simulink model "WMMSupportingForcesGP2021b"  (R2021b)
settings: Solver=ode23t  StartTime=0.0  StopTime=inf  FixedStep=.001  RelTol=1e-3  AbsTol=1e-3
InitFcn:
  | InitializeSimulationGP
  | SimulationParametersGP
values from neighbouring files (symbols this model uses):
  B11_r_B11C = [0.23805608; 0.13201777; 0]    [InitializeSimulationGP.m]
  B11_r_B11Tc1 = [L11; 0; 0]    [InitializeSimulationGP.m]
  B11_Rot_Tc1 = eye(3)    [InitializeSimulationGP.m]
  B11cI = [0.28426000 -0.06487287 0;         -0.06487287  0.54237481 0;                   0  0          0.67891020]    [InitializeSimulationGP.m]
  B12_r_B12C = [0.60504569; 0.27199376; 0.00002484]    [InitializeSimulationGP.m]
  B12_r_B12Tc2 = [L12;0;0]    [InitializeSimulationGP.m]
  B12_Rot_Tc2 = eye(3)    [InitializeSimulationGP.m]
  B12cI = [1.18803886 -2.36786418 0.00280315;          -2.36786418 6.31493281 0.00022322;           0.00280315 0.00022322 7.40915161]    [InitializeSimulationGP.m]
  B31_r_B31C = [0.35781210 0 0]    [InitializeSimulationGP.m]
  B31_Rot_B41 = eye(3)    [InitializeSimulationGP.m]
  B31cI = diag([0.03150902 0.90735702 0.90763033])    [InitializeSimulationGP.m]
  B32_r_B32C = [0.35781210 0 0]    [InitializeSimulationGP.m]
  B32_Rot_B42 = eye(3)    [InitializeSimulationGP.m]
  B32cI = diag([0.03150902 0.90735702 0.90763033])    [InitializeSimulationGP.m]
  B41_r_B41C = [0.55785997 0 0]    [InitializeSimulationGP.m]
  B41_r_B41Tc1 = [lc1;0;0]    [InitializeSimulationGP.m]
  B41cI = diag([0.00370720 0.55759812 0.55785997])    [InitializeSimulationGP.m]
  B42_r_B42C = [0.55785997 0 0]    [InitializeSimulationGP.m]
  B42_r_B42Tc2 = [lc2; 0; 0]    [InitializeSimulationGP.m]
  B42cI = diag([0.00370720 0.55759812 0.55785997])    [InitializeSimulationGP.m]
  B52_r_B52C = [0 0 0.56802906]    [InitializeSimulationGP.m]
  B52_r_B52P32 = [lc3; 0; 0]    [InitializeSimulationGP.m]
  B52_Rot_P32 = eye(3)    [InitializeSimulationGP.m]
  B52cI = diag([0.91789884, 0.91790043, 0.00091463])    [InitializeSimulationGP.m]
  Bc1_r_Bc1B11 = [L1; 0; 0]    [InitializeSimulationGP.m]
  Bc1_r_Bc1B31 = [0;0;0]    [InitializeSimulationGP.m]
  Bc1_r_Bc1C = [0.14178771; 0.16555780; 0]    [InitializeSimulationGP.m]
  Bc1_V = [0;0;0;0;0;0]    [InitializeSimulationGP.m]
  Bc1cI = [+5.892211080 +5.476111360 -0.000019630;          +5.476111360 +28.66965601 -0.000024550;          -0.000019630 -0.000024550 +29.78955950]    [InitializeSimulationGP.m]
  Bc2_r_Bc2B12 = [L2;0;0]    [InitializeSimulationGP.m]
  Bc2_r_Bc2B32 = [0;0;0]    [InitializeSimulationGP.m]
  Bc2_r_Bc2C = [0.54319901; 0.10543875; 0]    [InitializeSimulationGP.m]
  Bc2cI = [0.48071390 0.52924041 0;          0.52924041 5.80912352 0;              0      0          5.97255351]    [InitializeSimulationGP.m]
  BC_r_BCBM = [xCA; yCA; zCA]    [SimulationParametersGP.m]
  BC_Rot_BM = eye(3)    [SimulationParametersGP.m]
  BCI = diag([100 1200 1000])    [SimulationParametersGP.m]
  beta1 = atan2d(374.261,935)*pi/180    [InitializeSimulationGP.m]
  beta2 = atan2d(45.757,373.313)*pi/180    [InitializeSimulationGP.m]
  beta3 = atan2d(139.50,1132.19)*pi/180    [InitializeSimulationGP.m]
  beta4 = atan2d(88.061,296.198)*pi/180    [InitializeSimulationGP.m]
  betaGround = 1e6    (= 1000000)    [SimulationParametersGP.m]
  BFL = 0.05    [SimulationParametersGP.m]
  BFR = 0.05    [SimulationParametersGP.m]
  BM_r_BMBMp = [0;0;0]    [SimulationParametersGP.m]
  BM_Rot_BMp = [cos(gamma) -sin(gamma) 0; sin(gamma) cos(gamma) 0; 0 0 1]    [SimulationParametersGP.m]
  BMp_r_BMpBc1 = [0.185;0;0.205]    [InitializeSimulationGP.m]
  BMp_Rot_Bc1 = [cos(alpha1) -sin(alpha1)  0;                  0            0       -1;                sin(alpha1)  cos(alpha1)  0]    [InitializeSimulationGP.m]
  BRL = 0.05    [SimulationParametersGP.m]
  BRR = 0.05    [SimulationParametersGP.m]
  cc = 0.0    (= 0)    [SimulationParametersGP.m]
  D22F = [0;0;0;0;0;0]    [InitializeSimulationGP.m]
  dT = 0.01    [SimulationParametersGP.m]
  g0 = 9.8066    [SimulationParametersGP.m]
  ground_stiffness = 1e8    (= 100000000)    [SimulationParametersGP.m]
  l1 = 1.15-cc    (= 1.15)    [SimulationParametersGP.m]
  L1 = 1.0071227324212    (= 1.00712273242)    [InitializeSimulationGP.m]
  L11 = 0.37610632101293    (= 0.376106321013)    [InitializeSimulationGP.m]
  L12 = 0.30901132665325    (= 0.309011326653)    [InitializeSimulationGP.m]
  l2 = 1.15+cc    (= 1.15)    [SimulationParametersGP.m]
  L2 = 1.132185817991    (= 1.13218581799)    [InitializeSimulationGP.m]
  lc1 = 0.745    [InitializeSimulationGP.m]
  lc2 = 0.745    [InitializeSimulationGP.m]
  mB11 = 25.52660174    [InitializeSimulationGP.m]
  mB12 = 33.92850233    [InitializeSimulationGP.m]
  mB31 = 17.36281648    [InitializeSimulationGP.m]
  mB32 = 17.36281648    [InitializeSimulationGP.m]
  mB41 = 10.34519231    [InitializeSimulationGP.m]
  mB42 = 10.34519231    [InitializeSimulationGP.m]
  mB52 = 6.73059863    [InitializeSimulationGP.m]
  mBC = 2200    [SimulationParametersGP.m]
  mBc1 = 307.29601379    [InitializeSimulationGP.m]
  mBc2 = 54.58702836    [InitializeSimulationGP.m]
  mFL = 60    [SimulationParametersGP.m]
  mFR = 60    [SimulationParametersGP.m]
  mP22 = 9.26136143    [InitializeSimulationGP.m]
  mP32 = 570.18877059    [InitializeSimulationGP.m]
  mRR = 60    [SimulationParametersGP.m]
  mw = mFL    (= 60)    [SimulationParametersGP.m]
  P22_r_P22C = [0.62192523 0 0]    [InitializeSimulationGP.m]
  P22_Rot_B52 = eye(3)    [InitializeSimulationGP.m]
  P22cI = diag([0.00662754, 1.48387017, 1.48398069])    [InitializeSimulationGP.m]
  P32_r_P32C = [0.25466704; -0.13034397; -0.01302248]    [InitializeSimulationGP.m]
  P32_r_P32D22 = [0.40499744871392; -0.13130517281345; -0.013385243295654]    [InitializeSimulationGP.m]
  P32_Rot_D22 = [1 0 0;              0 0.9707729441837 0.23999977258512;              0 -0.23999977258512 0.9707729441837]    [InitializeSimulationGP.m]
  P32cI = [46.81220713 0.38607676 -0.00453819;          0.38607676 71.92201786 -1.14320993;          -0.00453819 -1.14320993 67.38128576]    [InitializeSimulationGP.m]
  R0FL = 0.35    [SimulationParametersGP.m]
  R0FR = 0.35    [SimulationParametersGP.m]
  R0RL = 0.35    [SimulationParametersGP.m]
  R0RR = 0.35    [SimulationParametersGP.m]
  Rw = R0FL    (= 0.35)    [SimulationParametersGP.m]
  Tc1_r_Tc1Bc2 = [0.098495302558553; 0.01838181329939; 0]    [InitializeSimulationGP.m]
  Tc1_Rot_Bc2 = [cos(alpha2) -sin(alpha2) 0;                sin(alpha2)  cos(alpha2) 0;                0            0           1]    [InitializeSimulationGP.m]
  Tc2_r_Tc2P22 = [-0.048858374920227;0.36587359346146;0.035276938723102]    [InitializeSimulationGP.m]
  Tc2_Rot_P22 = [0.95853460763586 -0.27664713597974  0.0683942111482;                0.28497614981675  0.93051946315663 -0.23004808784757;                0                 0.23999977258511  0.9707729441837]    [InitializeSimulationGP.m]
  Th1A = 10*pi/180    (= 0.174532925199)    [InitializeSimulationGP.m]
  Th1B = 20*pi/180    (= 0.349065850399)    [InitializeSimulationGP.m]
  Th1f = 1    [InitializeSimulationGP.m]
  Th2A = 15*pi/180    (= 0.261799387799)    [InitializeSimulationGP.m]
  Th2B = -70*pi/180    (= -1.2217304764)    [InitializeSimulationGP.m]
  Th2f = 2    [InitializeSimulationGP.m]
  w = wFL    (= 0.875)    [SimulationParametersGP.m]
  W_r_WBc1 = [0.185;0;0.205]    [InitializeSimulationGP.m]
  W_Rot_Bc1 = [cos(alpha1) -sin(alpha1)  0;                  0            0       -1;                sin(alpha1)  cos(alpha1)  0]    [InitializeSimulationGP.m]
  x10 = 0.83    [InitializeSimulationGP.m]
  x20 = 0.83    [InitializeSimulationGP.m]
  x3A = 0.2    [InitializeSimulationGP.m]
  x3B = 0.3    [InitializeSimulationGP.m]
  x3f = 1    [InitializeSimulationGP.m]
  xCA = 0.5    [SimulationParametersGP.m]
  xf = [1;0;0;0;0;0]    [InitializeSimulationGP.m]
  yCA = 0    [SimulationParametersGP.m]
  zC = 0.45    [SimulationParametersGP.m]
  zCA = .25    (= 0.25)    [SimulationParametersGP.m]
  ztau = [0;0;0;0;0;1]    [InitializeSimulationGP.m]
undefined symbols (not defined in the file or in its folder): alphaFL_meas, alphaFR_meas, alphaRL_meas, alphaRR_meas, B11_V, B11Ftot, B12_U_Tc2, B12_V, B12Ftot, B31_r_B31B41, B31_V, B31FTot, B32_r_B32B42, B32_U_B42, B32_V, B32FTot, B41_V, B41FTot, B42_Rot_Tc2, B42_U_Tc2, B42_V, B42FTot, B52_U_P32, B52_V, B52Ftot, Bc1Tot, Bc2_Rot_B12, Bc2_Rot_B32, Bc2_U_B12, Bc2_U_B32, Bc2_V, Bc2Tot, betaC_meas, D22_V, deltaFL_cmd, deltaFL_meas, deltaFR_cmd, deltaFR_meas, deltaRL_cmd, deltaRL_meas, deltaRR_cmd, deltaRR_meas, dOmegaFL_meas, dOmegaFR_meas, dOmegaRL_meas, dOmegaRR_meas, dPsi_meas, dq1, dq11, dq12, dq2, dq21, dq22, dx1, dx2, Floor, FTot_S1, FTot_S2P, FTot_S2R, FzFL ... (+63)
libraries: sm_lib x94, nesl_utility x63, simulink x5
(part 2 of 11)

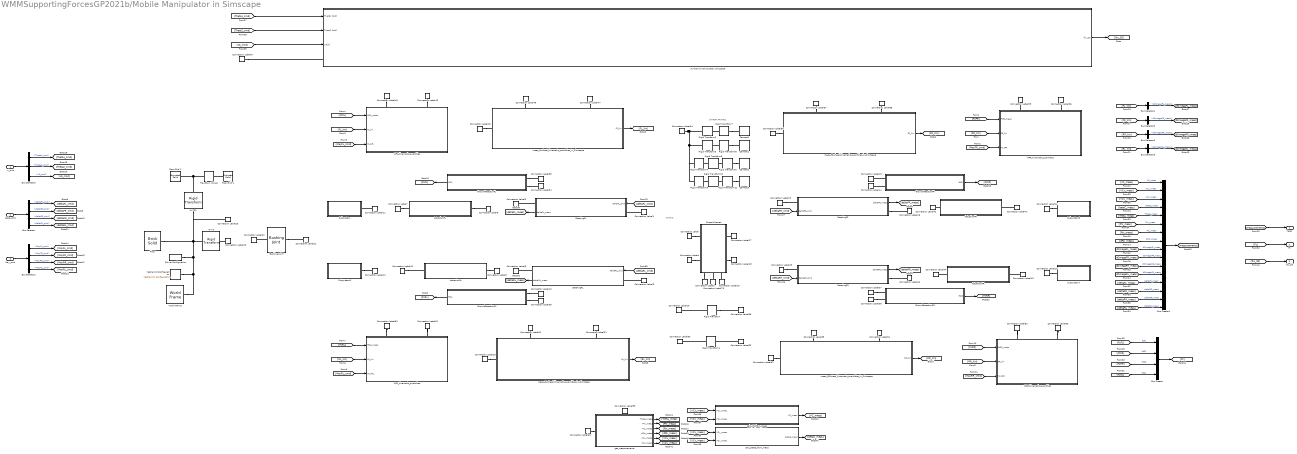
== system WMMSupportingForcesGP2021b/Mobile Manipulator in Simscape ==
  note: CAMERA FRAMES
  note: CHASIS
  xi_cmd : Inport
  delta_cmd : Inport  Port=2
  May_cmd : Inport  Port=3
  ActuationFL : Subsystem
  ActuationFR : Subsystem
  ActuationRL : Subsystem
  ActuationRR : Subsystem
  Bus Creator : BusCreator  Inputs=FzFL,FzFR,FzRR,FzRL
  Bus Creator1 : BusCreator  Inputs=VC_meas,VCx_meas,VCy_meas,betaC_meas,Theta_meas,Phi_meas,Psi_meas,dPsi_meas,dOmegaFL_meas,dOmegaFR_meas,dOmegaRR_meas,dOmegaRL_meas,deltaFL_meas,deltaFR_meas,deltaRR_meas,deltaRL_meas
  Bus Selector : BusSelector  OutputSignals=deltaFL_cmd,deltaFR_cmd,deltaRR_cmd,deltaRL_cmd
  Bus Selector1 : BusSelector  OutputSignals=MayFL_cmd,MayFR_cmd,MayRR_cmd,MayRL_cmd
  Bus Selector2 : BusSelector  OutputSignals=Theta1_cmd,Theta2_cmd,x3_cmd
  Bus Selector3 : BusSelector  OutputSignals=dOmegaFR_meas
  Bus Selector4 : BusSelector  OutputSignals=dOmegaFL_meas
  Bus Selector5 : BusSelector  OutputSignals=dOmegaRR_meas
  Bus Selector6 : BusSelector  OutputSignals=dOmegaRL_meas
  Bushing Joint : sm_lib/Joints/Bushing Joint  JointMode=Normal  SenseConstraintForce=off  SenseConstraintForceX=off  SenseConstraintForceY=off  SenseConstraintForceZ=off  SenseConstraintTorque=off  SenseConstraintTorqueX=off  SenseConstraintTorqueY=off  SenseConstraintTorqueZ=off  SenseTotalForce=off  SenseTotalForceX=off  SenseTotalForceY=off  SenseTotalForceZ=off  SenseTotalTorque=off  SenseTotalTorqueX=off  SenseTotalTorqueY=off  SenseTotalTorqueZ=off  CompositeWrenchDir=FollowerOnBase  CompositeWrenchFrame=BaseFrame  PxEquilibriumPosition=0  PxEquilibriumPositionUnits=m  PxSpringStiffness=0  PxSpringStiffnessUnits=N/m  PxDampingCoefficient=0  PxDampingCoefficientUnits=N/(m/s)  PxTorqueActuationMode=NoTorque  PxMotionActuationMode=ComputedMotion  PxSensePosition=off  PxSenseVelocity=off  PxSenseAcceleration=off  PxSenseTorqueForce=off  PxSenseLowerLimitTorqueForce=off  PxSenseUpperLimitTorqueForce=off  PxLowerLimitSpecify=off  PxLowerLimitBound=-1  PxLowerLimitBoundUnits=m  PxLowerLimitStiffness=1e6  PxLowerLimitStiffnessUnits=N/m  PxLowerLimitDamping=1e3  PxLowerLimitDampingUnits=N/(m/s)  PxLowerLimitTransitionRegionWidth=1e-4  PxLowerLimitTransitionRegionWidthUnits=m  PxUpperLimitSpecify=off  PxUpperLimitBound=1  PxUpperLimitBoundUnits=m  PxUpperLimitStiffness=1e6  PxUpperLimitStiffnessUnits=N/m  PxUpperLimitDamping=1e3  PxUpperLimitDampingUnits=N/(m/s)  PxUpperLimitTransitionRegionWidth=1e-4  PxUpperLimitTransitionRegionWidthUnits=m  PxPositionTargetSpecify=off  PxPositionTargetPriority=High  PxPositionTargetValue=0  PxPositionTargetValueUnits=m  PxVelocityTargetSpecify=off  PxVelocityTargetPriority=High  PxVelocityTargetValue=0  PxVelocityTargetValueUnits=m/s  PyEquilibriumPosition=0  PyEquilibriumPositionUnits=m  PySpringStiffness=0  PySpringStiffnessUnits=N/m  PyDampingCoefficient=0  PyDampingCoefficientUnits=N/(m/s)  PyTorqueActuationMode=NoTorque  PyMotionActuationMode=ComputedMotion  PySensePosition=off  PySenseVelocity=off  PySenseAcceleration=off  PySenseTorqueForce=off  PySenseLowerLimitTorqueForce=off  PySenseUpperLimitTorqueForce=off  PyLowerLimitSpecify=off  PyLowerLimitBound=-1  PyLowerLimitBoundUnits=m  PyLowerLimitStiffness=1e6  PyLowerLimitStiffnessUnits=N/m  PyLowerLimitDamping=1e3  PyLowerLimitDampingUnits=N/(m/s)  PyLowerLimitTransitionRegionWidth=1e-4  PyLowerLimitTransitionRegionWidthUnits=m  PyUpperLimitSpecify=off  PyUpperLimitBound=1  PyUpperLimitBoundUnits=m  PyUpperLimitStiffness=1e6  PyUpperLimitStiffnessUnits=N/m  PyUpperLimitDamping=1e3  PyUpperLimitDampingUnits=N/(m/s)  PyUpperLimitTransitionRegionWidth=1e-4  PyUpperLimitTransitionRegionWidthUnits=m  PyPositionTargetSpecify=off  PyPositionTargetPriority=High  PyPositionTargetValue=0  PyPositionTargetValueUnits=m  PyVelocityTargetSpecify=off  PyVelocityTargetPriority=High  PyVelocityTargetValue=0  PyVelocityTargetValueUnits=m/s  PzEquilibriumPosition=0  PzEquilibriumPositionUnits=m  PzSpringStiffness=0  PzSpringStiffnessUnits=N/m  PzDampingCoefficient=0  PzDampingCoefficientUnits=N/(m/s)  PzTorqueActuationMode=NoTorque  PzMotionActuationMode=ComputedMotion  PzSensePosition=off  PzSenseVelocity=off  PzSenseAcceleration=off  PzSenseTorqueForce=off  PzSenseLowerLimitTorqueForce=off  PzSenseUpperLimitTorqueForce=off  PzLowerLimitSpecify=off  PzLowerLimitBound=-1  PzLowerLimitBoundUnits=m  PzLowerLimitStiffness=1e6  PzLowerLimitStiffnessUnits=N/m  PzLowerLimitDamping=1e3  PzLowerLimitDampingUnits=N/(m/s)  PzLowerLimitTransitionRegionWidth=1e-4  PzLowerLimitTransitionRegionWidthUnits=m  PzUpperLimitSpecify=off  PzUpperLimitBound=1  PzUpperLimitBoundUnits=m  PzUpperLimitStiffness=1e6  PzUpperLimitStiffnessUnits=N/m  PzUpperLimitDamping=1e3  PzUpperLimitDampingUnits=N/(m/s)  PzUpperLimitTransitionRegionWidth=1e-4  PzUpperLimitTransitionRegionWidthUnits=m  PzPositionTargetSpecify=off  PzPositionTargetPriority=High  PzPositionTargetValue=0  PzPositionTargetValueUnits=m  PzVelocityTargetSpecify=off  PzVelocityTargetPriority=High  PzVelocityTargetValue=0  PzVelocityTargetValueUnits=m/s  RxEquilibriumPosition=0  RxEquilibriumPositionUnits=deg  RxSpringStiffness=0  RxSpringStiffnessUnits=N*m/deg  RxDampingCoefficient=0  RxDampingCoefficientUnits=N*m/(deg/s)  RxTorqueActuationMode=NoTorque  RxMotionActuationMode=ComputedMotion  RxSensePosition=off  RxSenseVelocity=off  RxSenseAcceleration=off  RxSenseTorqueForce=off  RxSenseLowerLimitTorqueForce=off  RxSenseUpperLimitTorqueForce=off  RxLowerLimitSpecify=off  RxLowerLimitBound=-90  RxLowerLimitBoundUnits=deg  RxLowerLimitStiffness=1e4  RxLowerLimitStiffnessUnits=N*m/deg  RxLowerLimitDamping=10  RxLowerLimitDampingUnits=N*m/(deg/s)  RxLowerLimitTransitionRegionWidth=0.1  RxLowerLimitTransitionRegionWidthUnits=deg  RxUpperLimitSpecify=off  RxUpperLimitBound=90  RxUpperLimitBoundUnits=deg  RxUpperLimitStiffness=1e4  RxUpperLimitStiffnessUnits=N*m/deg  RxUpperLimitDamping=10  RxUpperLimitDampingUnits=N*m/(deg/s)  RxUpperLimitTransitionRegionWidth=0.1  RxUpperLimitTransitionRegionWidthUnits=deg  RxPositionTargetSpecify=off  RxPositionTargetPriority=High  RxPositionTargetValue=0  RxPositionTargetValueUnits=deg  RxVelocityTargetSpecify=off  RxVelocityTargetPriority=High  RxVelocityTargetValue=0  RxVelocityTargetValueUnits=deg/s  RyEquilibriumPosition=0  RyEquilibriumPositionUnits=deg  RySpringStiffness=0  RySpringStiffnessUnits=N*m/deg  RyDampingCoefficient=0  RyDampingCoefficientUnits=N*m/(deg/s)  RyTorqueActuationMode=NoTorque  RyMotionActuationMode=ComputedMotion  RySensePosition=off  RySenseVelocity=off  RySenseAcceleration=off  RySenseTorqueForce=off  RySenseLowerLimitTorqueForce=off  RySenseUpperLimitTorqueForce=off  RyLowerLimitSpecify=off  RyLowerLimitBound=-90  RyLowerLimitBoundUnits=deg  RyLowerLimitStiffness=1e4  RyLowerLimitStiffnessUnits=N*m/deg  RyLowerLimitDamping=10  RyLowerLimitDampingUnits=N*m/(deg/s)  RyLowerLimitTransitionRegionWidth=0.1  RyLowerLimitTransitionRegionWidthUnits=deg  RyUpperLimitSpecify=off  RyUpperLimitBound=90  RyUpperLimitBoundUnits=deg  RyUpperLimitStiffness=1e4  RyUpperLimitStiffnessUnits=N*m/deg  RyUpperLimitDamping=10  RyUpperLimitDampingUnits=N*m/(deg/s)  RyUpperLimitTransitionRegionWidth=0.1  RyUpperLimitTransitionRegionWidthUnits=deg  RyPositionTargetSpecify=off  RyPositionTargetPriority=High  RyPositionTargetValue=0  RyPositionTargetValueUnits=deg  RyVelocityTargetSpecify=off  RyVelocityTargetPriority=High  RyVelocityTargetValue=0  RyVelocityTargetValueUnits=deg/s  RzEquilibriumPosition=0  RzEquilibriumPositionUnits=deg  RzSpringStiffness=0  RzSpringStiffnessUnits=N*m/deg  RzDampingCoefficient=0  RzDampingCoefficientUnits=N*m/(deg/s)  RzTorqueActuationMode=NoTorque  RzMotionActuationMode=ComputedMotion  RzSensePosition=off  RzSenseVelocity=off  RzSenseAcceleration=off  RzSenseTorqueForce=off  RzSenseLowerLimitTorqueForce=off  RzSenseUpperLimitTorqueForce=off  RzLowerLimitSpecify=off  RzLowerLimitBound=-90  RzLowerLimitBoundUnits=deg  RzLowerLimitStiffness=1e4  RzLowerLimitStiffnessUnits=N*m/deg  RzLowerLimitDamping=10  RzLowerLimitDampingUnits=N*m/(deg/s)  RzLowerLimitTransitionRegionWidth=0.1  RzLowerLimitTransitionRegionWidthUnits=deg  RzUpperLimitSpecify=off  RzUpperLimitBound=90  RzUpperLimitBoundUnits=deg  RzUpperLimitStiffness=1e4  RzUpperLimitStiffnessUnits=N*m/deg  RzUpperLimitDamping=10  RzUpperLimitDampingUnits=N*m/(deg/s)  RzUpperLimitTransitionRegionWidth=0.1  RzUpperLimitTransitionRegionWidthUnits=deg  RzPositionTargetSpecify=off  RzPositionTargetPriority=High  RzPositionTargetValue=0  RzPositionTargetValueUnits=deg  RzVelocityTargetSpecify=off  RzVelocityTargetPriority=High  RzVelocityTargetValue=0  RzVelocityTargetValueUnits=deg/s
  Camera{0..3} (4 alike) : sm_lib/Frames and Transforms/Reference Frame
  Chassis frames : Subsystem
      settings: PortSchema="{\"entries\":[{\"content\":{\"sides\":[{\"content\":{\"connectorIds\":[\"LConn1\",\"LConn2\"]},\"type\":\"ConnectorPlacement.EquallySpacedRectSide\",\"uuid\":\"eef62e1d-15c3-48f9-a200-1ec7cba34bfd\"},{\"content\":{\"connectorIds\":[\"RConn1\",\"RConn2\"],\"side\":\"RIGHT\"},\"type\":\"ConnectorPlacement.EquallySpacedRectSide\",\"uuid\":\"68cd7829-07b7-4c33-9669-dcec97cc4467\"},{\"content\":{\"connectorIds\":[],\"side\":\"TOP\"},\"type\":\"ConnectorPlacement.EquallySpacedRectSide\",\"uuid\":\"a2020256-aba7-4d86-a2a6-b0271002a0c7\"},{\"content\":{\"connectorIds\":[\"RConn3\",\"RConn4\",\"RConn5\"],\"side\":\"BOTTOM\"},\"type\":\"ConnectorPlacement.EquallySpacedRectSide\",\"uuid\":\"c369bc44-4007-4272-b5f0-3026cf2c22ef\"}]},\"type\":\"ConnectorPlacement.EquallySpacedConnector\",\"uuid\":\"d60cd83d-8810-499d-88ee-1107911897a7\"}],\"packageUris\":[\"http://schema.mathworks.com/mf0/Connector/R2020b\"],\"version\":\"1.0\"}"
  Connection Label : ConnectionLabel  Label=CFL
  Connection Label1 : ConnectionLabel  Label=CFL
  Connection Label{10,12,31,51} (4 alike) : ConnectionLabel  Label=WRLp
  Connection Label{7,11,47,49} (4 alike) : ConnectionLabel  Label=WFLp
  Connection Label{13,23,29,32,37,39,45,54,56,63} (10 alike) : ConnectionLabel  Label=W
  Connection Label{14,16,35,42,57} (5 alike) : ConnectionLabel  Label=WFR
  Connection Label15 : ConnectionLabel  Label=CFR
  Connection Label17 : ConnectionLabel  Label=CFR
  Connection Label18 : ConnectionLabel  Label=CRR
  Connection Label19 : ConnectionLabel  Label=B
  Connection Label2 : ConnectionLabel  Label=BC
  Connection Label20 : ConnectionLabel  Label=BC
  Connection Label21 : ConnectionLabel  Label=O
  Connection Label22 : ConnectionLabel  Label=S
  Connection Label{24,36,41,65} (4 alike) : ConnectionLabel  Label=WFRp
  Connection Label25 : ConnectionLabel  Label=CRR
  Connection Label{26,33,38,44,52} (5 alike) : ConnectionLabel  Label=WRR
  Connection Label{27,34,43,53} (4 alike) : ConnectionLabel  Label=WRRp
  Connection Label28 : ConnectionLabel  Label=S
  Connection Label3 : ConnectionLabel  Label=CRL
  Connection Label{6,9,30,40,50} (5 alike) : ConnectionLabel  Label=WRL
  Connection Label4 : ConnectionLabel  Label=CRL
  Connection Label{5,8,46,48,55} (5 alike) : ConnectionLabel  Label=WFL
  Connection Label58 : ConnectionLabel  Label=BM
  Connection Label59 : ConnectionLabel  Label=BC
  Connection Label60 : ConnectionLabel  Label=BM
  Connection Label62 : ConnectionLabel  Label=BMp
  Connection Label64 : ConnectionLabel  Label=BM
  Connection Label67 : ConnectionLabel  Label=BMp
  Connection Label75 : ConnectionLabel  Label=O
  Floor : sm_lib/Body Elements/Brick Solid  GraphicAmbientColor=[0.15 0.15 0.15 1.0]  BasedOnType=Density  BrickDimensions=[1000 1000 .1]  BrickDimensionUnits=m  CenterOfMass=[0 0 0]  CenterOfMassUnits=m  GraphicDiffuseColor=[0.8 1.0 0.8]  Density=1000  DensityUnits=kg/m^3  DoExposeReferenceFrame=off  GraphicEmissiveColor=[0.0 0.0 0.0 1.0]  ExportEntireGeometry=off  SerializedFrames=<Frames><Frame><Id>Frame2</Id><Value><Name>W</Name><Origin><Source>GeometricFeature</Source><FeatureName>+z -x curve</FeatureName></Origin><PrimaryAxis><DefinedDirection>+Z</DefinedDirection><Source>ReferenceFrame</Source><SourceDirection>+Z</SourceDirection><FeatureName></FeatureName></PrimaryAxis><SecondaryAxis><DefinedDirection>+X</DefinedDirection><Source>ReferenceFrame</Source><SourceDirection>+X</SourceDirection><FeatureName></FeatureName></SecondaryAxis></Value></Frame></Frames>  MarkerShape=Sphere  MarkerSize=10  GraphicType=FromGeometry  InertiaType=CalculateFromGeometry  Mass=1  MassUnits=kg  MomentsOfInertia=[1 1 1]  MomentsOfInertiaUnits=kg*m^2  GraphicOpacity=1  ProductsOfInertia=[0 0 0]  ProductsOfInertiaUnits=kg*m^2  GraphicShininess=75  GraphicSpecularColor=[0.5 0.5 0.5 1.0]  GraphicVisPropType=SimpleVisualProperties
  Floor Grid 1 : sm_lib/Body Elements/Extruded Solid  GraphicAmbientColor=[0.15 0.15 0.15 1.0]  BasedOnType=Density  CenterOfMass=[0 0 0]  CenterOfMassUnits=m  GraphicDiffuseColor=[1.0 0.2 0.4]  ExportConvexHullGeometry=off  ExtrusionCrossSection=Grid.extr_data  ExtrusionCrossSectionUnits=m  Density=1000  DensityUnits=kg/m^3  DoExposeReferenceFrame=on  GraphicEmissiveColor=[0.0 0.0 0.0 1.0]  ExportEntireGeometry=off  ExtrusionLength=Floor.h*1.005  ExtrusionLengthUnits=m  ExtrusionType=General  SerializedFrames=<Frames/>  MarkerShape=Sphere  MarkerSize=10  GraphicType=FromGeometry  InertiaType=PointMass  Mass=1  MassUnits=kg  MomentsOfInertia=[1 1 1]  MomentsOfInertiaUnits=kg*m^2  PolygonNumSides=3  GraphicOpacity=1.0  PolygonOuterRadius=1  PolygonOuterRadiusUnits=m  ProductsOfInertia=[1 1 1]  ProductsOfInertiaUnits=kg*m^2  GraphicShininess=75  GraphicSpecularColor=[0.5 0.5 0.5 1.0]  GraphicVisPropType=SimpleVisualProperties
  Floor Grid 2 : sm_lib/Body Elements/Extruded Solid  GraphicAmbientColor=[0.15 0.15 0.15 1.0]  BasedOnType=Density  CenterOfMass=[0 0 0]  CenterOfMassUnits=m  GraphicDiffuseColor=[1.0 0.0 0.2]  ExportConvexHullGeometry=off  ExtrusionCrossSection=Grid.extr_data  ExtrusionCrossSectionUnits=m  Density=1000  DensityUnits=kg/m^3  DoExposeReferenceFrame=on  GraphicEmissiveColor=[0.0 0.0 0.0 1.0]  ExportEntireGeometry=off  ExtrusionLength=Floor.h*1.005  ExtrusionLengthUnits=m  ExtrusionType=General  SerializedFrames=<Frames/>  MarkerShape=Sphere  MarkerSize=10  GraphicType=FromGeometry  InertiaType=PointMass  Mass=1  MassUnits=kg  MomentsOfInertia=[1 1 1]  MomentsOfInertiaUnits=kg*m^2  PolygonNumSides=3  GraphicOpacity=1.0  PolygonOuterRadius=1  PolygonOuterRadiusUnits=m  ProductsOfInertia=[1 1 1]  ProductsOfInertiaUnits=kg*m^2  GraphicShininess=75  GraphicSpecularColor=[0.5 0.5 0.5 1.0]  GraphicVisPropType=SimpleVisualProperties
  GroundReactionFL : Subsystem
      settings: PortSchema="{\"entries\":[{\"content\":{\"sides\":[{\"content\":{\"connectorIds\":[\"Out1\"]},\"type\":\"ConnectorPlacement.EquallySpacedRectSide\",\"uuid\":\"83a50a17-2c26-4437-a264-c8e6d16b5f5b\"},{\"content\":{\"connectorIds\":[\"RConn1\",\"RConn2\"],\"side\":\"RIGHT\"},\"type\":\"ConnectorPlacement.EquallySpacedRectSide\",\"uuid\":\"9399cf75-3dd9-45fa-85d6-db5b88096a02\"},{\"content\":{\"connectorIds\":[],\"side\":\"TOP\"},\"type\":\"ConnectorPlacement.EquallySpacedRectSide\",\"uuid\":\"59849b12-7527-4fe3-9ac1-a960d161aef4\"},{\"content\":{\"connectorIds\":[],\"side\":\"BOTTOM\"},\"type\":\"ConnectorPlacement.EquallySpacedRectSide\",\"uuid\":\"c578aa5d-499f-4dfc-8d0b-42fb5daa91e6\"}]},\"type\":\"ConnectorPlacement.EquallySpacedConnector\",\"uuid\":\"74a78a0d-1728-4273-b294-ce3cbd63255e\"}],\"packageUris\":[\"http://schema.mathworks.com/mf0/Connector/R2020b\"],\"version\":\"1.0\"}"
  GroundReactionFR : Subsystem
      settings: PortSchema="{\"entries\":[{\"content\":{\"sides\":[{\"content\":{\"connectorIds\":[\"Out1\"]},\"type\":\"ConnectorPlacement.EquallySpacedRectSide\",\"uuid\":\"83a50a17-2c26-4437-a264-c8e6d16b5f5b\"},{\"content\":{\"connectorIds\":[\"RConn1\",\"RConn2\"],\"side\":\"RIGHT\"},\"type\":\"ConnectorPlacement.EquallySpacedRectSide\",\"uuid\":\"9399cf75-3dd9-45fa-85d6-db5b88096a02\"},{\"content\":{\"connectorIds\":[],\"side\":\"TOP\"},\"type\":\"ConnectorPlacement.EquallySpacedRectSide\",\"uuid\":\"59849b12-7527-4fe3-9ac1-a960d161aef4\"},{\"content\":{\"connectorIds\":[],\"side\":\"BOTTOM\"},\"type\":\"ConnectorPlacement.EquallySpacedRectSide\",\"uuid\":\"c578aa5d-499f-4dfc-8d0b-42fb5daa91e6\"}]},\"type\":\"ConnectorPlacement.EquallySpacedConnector\",\"uuid\":\"74a78a0d-1728-4273-b294-ce3cbd63255e\"}],\"packageUris\":[\"http://schema.mathworks.com/mf0/Connector/R2020b\"],\"version\":\"1.0\"}"
  GroundReactionRL : Subsystem
      settings: PortSchema="{\"entries\":[{\"content\":{\"sides\":[{\"content\":{\"connectorIds\":[\"Out1\"]},\"type\":\"ConnectorPlacement.EquallySpacedRectSide\",\"uuid\":\"83a50a17-2c26-4437-a264-c8e6d16b5f5b\"},{\"content\":{\"connectorIds\":[\"RConn1\",\"RConn2\"],\"side\":\"RIGHT\"},\"type\":\"ConnectorPlacement.EquallySpacedRectSide\",\"uuid\":\"9399cf75-3dd9-45fa-85d6-db5b88096a02\"},{\"content\":{\"connectorIds\":[],\"side\":\"TOP\"},\"type\":\"ConnectorPlacement.EquallySpacedRectSide\",\"uuid\":\"59849b12-7527-4fe3-9ac1-a960d161aef4\"},{\"content\":{\"connectorIds\":[],\"side\":\"BOTTOM\"},\"type\":\"ConnectorPlacement.EquallySpacedRectSide\",\"uuid\":\"c578aa5d-499f-4dfc-8d0b-42fb5daa91e6\"}]},\"type\":\"ConnectorPlacement.EquallySpacedConnector\",\"uuid\":\"74a78a0d-1728-4273-b294-ce3cbd63255e\"}],\"packageUris\":[\"http://schema.mathworks.com/mf0/Connector/R2020b\"],\"version\":\"1.0\"}"
  GroundReactionRR : Subsystem
      settings: PortSchema="{\"entries\":[{\"content\":{\"sides\":[{\"content\":{\"connectorIds\":[\"Out1\"]},\"type\":\"ConnectorPlacement.EquallySpacedRectSide\",\"uuid\":\"83a50a17-2c26-4437-a264-c8e6d16b5f5b\"},{\"content\":{\"connectorIds\":[\"RConn1\",\"RConn2\"],\"side\":\"RIGHT\"},\"type\":\"ConnectorPlacement.EquallySpacedRectSide\",\"uuid\":\"9399cf75-3dd9-45fa-85d6-db5b88096a02\"},{\"content\":{\"connectorIds\":[],\"side\":\"TOP\"},\"type\":\"ConnectorPlacement.EquallySpacedRectSide\",\"uuid\":\"59849b12-7527-4fe3-9ac1-a960d161aef4\"},{\"content\":{\"connectorIds\":[],\"side\":\"BOTTOM\"},\"type\":\"ConnectorPlacement.EquallySpacedRectSide\",\"uuid\":\"c578aa5d-499f-4dfc-8d0b-42fb5daa91e6\"}]},\"type\":\"ConnectorPlacement.EquallySpacedConnector\",\"uuid\":\"74a78a0d-1728-4273-b294-ce3cbd63255e\"}],\"packageUris\":[\"http://schema.mathworks.com/mf0/Connector/R2020b\"],\"version\":\"1.0\"}"
  "Hydraulic manipulator, Simscape" : Subsystem
  MechanismConfiguration : sm_lib/Utilities/Mechanism Configuration  UniformGravity=Constant  GravityVector=[0 0 -9.8066]  GravityUnits=m/s^2  LinearizationDelta=0.001  JointModeTransitionNonlinearIterations=2
  Rigid Transform : sm_lib/Frames and Transforms/Rigid Transform  TranslationMethod=Cartesian  TranslationStandardOffset=0.3  TranslationLengthUnit=m  TranslationStandardAxis=+X  TranslationCartesianOffset=[xCA yCA zCA]  TranslationROffset=0  TranslationROffsetUnits=m  TranslationZOffset=0  TranslationZOffsetUnits=m  TranslationThetaOffset=0  TranslationThetaOffsetUnits=deg  RotationMethod=StandardAxis  RotationAngleUnits=deg  RotationStandardAxis=+Z  RotationAngle=0  RotationArbitraryAxis=[0 0 1]  FollAlignAxisA=+X  BaseAlignAxisA=+Y  FollAlignAxisB=+Y  BaseAlignAxisB=+Z  RotationSequenceAxes=FollowerAxes  RotationSequence=XYX  RotationSequenceAngles=[0 0 0]  RotationSequenceAnglesUnits=deg  RotationMatrix=[1 0 0; 0 1 0; 0 0 1]
  Rigid Transform1 : sm_lib/Frames and Transforms/Rigid Transform  TranslationMethod=None  TranslationStandardOffset=0  TranslationLengthUnit=m  TranslationStandardAxis=+Z  TranslationCartesianOffset=[0 0 0]  TranslationROffset=0  TranslationROffsetUnits=m  TranslationZOffset=0  TranslationZOffsetUnits=m  TranslationThetaOffset=0  TranslationThetaOffsetUnits=deg  RotationMethod=StandardAxis  RotationAngleUnits=rad  RotationStandardAxis=+Z  RotationAngle=gamma  RotationArbitraryAxis=[0 0 1]  FollAlignAxisA=+X  BaseAlignAxisA=+Y  FollAlignAxisB=+Y  BaseAlignAxisB=+Z  RotationSequenceAxes=FollowerAxes  RotationSequence=XYX  RotationSequenceAngles=[0 0 0]  RotationSequenceAnglesUnits=deg  RotationMatrix=[1 0 0; 0 1 0; 0 0 1]
  Rigid Transform10 : sm_lib/Frames and Transforms/Rigid Transform  TranslationMethod=None  TranslationStandardOffset=-10  TranslationLengthUnit=m  TranslationStandardAxis=+Y  TranslationCartesianOffset=[0 0 0]  TranslationROffset=0  TranslationROffsetUnits=m  TranslationZOffset=0  TranslationZOffsetUnits=m  TranslationThetaOffset=0  TranslationThetaOffsetUnits=deg  RotationMethod=StandardAxis  RotationAngleUnits=deg  RotationStandardAxis=+Z  RotationAngle=20  RotationArbitraryAxis=[0 0 1]  FollAlignAxisA=+X  BaseAlignAxisA=+Y  FollAlignAxisB=+Y  BaseAlignAxisB=+Z  RotationSequenceAxes=FollowerAxes  RotationSequence=XYX  RotationSequenceAngles=[0 0 0]  RotationSequenceAnglesUnits=deg  RotationMatrix=[1 0 0; 0 1 0; 0 0 1]
  Rigid Transform11 : sm_lib/Frames and Transforms/Rigid Transform  TranslationMethod=None  TranslationStandardOffset=-10  TranslationLengthUnit=m  TranslationStandardAxis=+Y  TranslationCartesianOffset=[0 0 0]  TranslationROffset=0  TranslationROffsetUnits=m  TranslationZOffset=0  TranslationZOffsetUnits=m  TranslationThetaOffset=0  TranslationThetaOffsetUnits=deg  RotationMethod=StandardAxis  RotationAngleUnits=deg  RotationStandardAxis=+Y  RotationAngle=20  RotationArbitraryAxis=[0 0 1]  FollAlignAxisA=+X  BaseAlignAxisA=+Y  FollAlignAxisB=+Y  BaseAlignAxisB=+Z  RotationSequenceAxes=FollowerAxes  RotationSequence=XYX  RotationSequenceAngles=[0 0 0]  RotationSequenceAnglesUnits=deg  RotationMatrix=[1 0 0; 0 1 0; 0 0 1]
  Rigid Transform2 : sm_lib/Frames and Transforms/Rigid Transform  TranslationMethod=Cartesian  TranslationStandardOffset=7  TranslationLengthUnit=m  TranslationStandardAxis=+X  TranslationCartesianOffset=[10 0 5]  TranslationROffset=0  TranslationROffsetUnits=m  TranslationZOffset=0  TranslationZOffsetUnits=m  TranslationThetaOffset=0  TranslationThetaOffsetUnits=deg  RotationMethod=None  RotationAngleUnits=deg  RotationStandardAxis=+Z  RotationAngle=0.0  RotationArbitraryAxis=[0 0 1]  FollAlignAxisA=+X  BaseAlignAxisA=+Y  FollAlignAxisB=+Y  BaseAlignAxisB=+Z  RotationSequenceAxes=FollowerAxes  RotationSequence=XYX  RotationSequenceAngles=[0 0 0]  RotationSequenceAnglesUnits=deg  RotationMatrix=[1 0 0; 0 1 0; 0 0 1]
  Rigid Transform3 : sm_lib/Frames and Transforms/Rigid Transform  TranslationMethod=Cartesian  TranslationStandardOffset=-10  TranslationLengthUnit=m  TranslationStandardAxis=+X  TranslationCartesianOffset=[-10 0 5]  TranslationROffset=0  TranslationROffsetUnits=m  TranslationZOffset=0  TranslationZOffsetUnits=m  TranslationThetaOffset=0  TranslationThetaOffsetUnits=deg  RotationMethod=None  RotationAngleUnits=deg  RotationStandardAxis=+Z  RotationAngle=0.0  RotationArbitraryAxis=[0 0 1]  FollAlignAxisA=+X  BaseAlignAxisA=+Y  FollAlignAxisB=+Y  BaseAlignAxisB=+Z  RotationSequenceAxes=FollowerAxes  RotationSequence=XYX  RotationSequenceAngles=[0 0 0]  RotationSequenceAnglesUnits=deg  RotationMatrix=[1 0 0; 0 1 0; 0 0 1]
  Rigid Transform4 : sm_lib/Frames and Transforms/Rigid Transform  TranslationMethod=Cartesian  TranslationStandardOffset=-10  TranslationLengthUnit=m  TranslationStandardAxis=+X  TranslationCartesianOffset=[-10 10 10]  TranslationROffset=0  TranslationROffsetUnits=m  TranslationZOffset=0  TranslationZOffsetUnits=m  TranslationThetaOffset=0  TranslationThetaOffsetUnits=deg  RotationMethod=None  RotationAngleUnits=deg  RotationStandardAxis=+Z  RotationAngle=0.0  RotationArbitraryAxis=[0 0 1]  FollAlignAxisA=+X  BaseAlignAxisA=+Y  FollAlignAxisB=+Y  BaseAlignAxisB=+Z  RotationSequenceAxes=FollowerAxes  RotationSequence=XYX  RotationSequenceAngles=[0 0 0]  RotationSequenceAnglesUnits=deg  RotationMatrix=[1 0 0; 0 1 0; 0 0 1]
  Rigid Transform5 : sm_lib/Frames and Transforms/Rigid Transform  TranslationMethod=None  TranslationStandardOffset=-10  TranslationLengthUnit=m  TranslationStandardAxis=+Y  TranslationCartesianOffset=[0 0 0]  TranslationROffset=0  TranslationROffsetUnits=m  TranslationZOffset=0  TranslationZOffsetUnits=m  TranslationThetaOffset=0  TranslationThetaOffsetUnits=deg  RotationMethod=StandardAxis  RotationAngleUnits=deg  RotationStandardAxis=-Z  RotationAngle=20  RotationArbitraryAxis=[0 0 1]  FollAlignAxisA=+X  BaseAlignAxisA=+Y  FollAlignAxisB=+Y  BaseAlignAxisB=+Z  RotationSequenceAxes=FollowerAxes  RotationSequence=XYX  RotationSequenceAngles=[0 0 0]  RotationSequenceAnglesUnits=deg  RotationMatrix=[1 0 0; 0 1 0; 0 0 1]
  Rigid Transform6 : sm_lib/Frames and Transforms/Rigid Transform  TranslationMethod=None  TranslationStandardOffset=-10  TranslationLengthUnit=m  TranslationStandardAxis=+Y  TranslationCartesianOffset=[0 0 0]  TranslationROffset=0  TranslationROffsetUnits=m  TranslationZOffset=0  TranslationZOffsetUnits=m  TranslationThetaOffset=0  TranslationThetaOffsetUnits=deg  RotationMethod=StandardAxis  RotationAngleUnits=deg  RotationStandardAxis=+Y  RotationAngle=20  RotationArbitraryAxis=[0 0 1]  FollAlignAxisA=+X  BaseAlignAxisA=+Y  FollAlignAxisB=+Y  BaseAlignAxisB=+Z  RotationSequenceAxes=FollowerAxes  RotationSequence=XYX  RotationSequenceAngles=[0 0 0]  RotationSequenceAnglesUnits=deg  RotationMatrix=[1 0 0; 0 1 0; 0 0 1]
  Rigid Transform7 : sm_lib/Frames and Transforms/Rigid Transform  TranslationMethod=None  TranslationStandardOffset=-10  TranslationLengthUnit=m  TranslationStandardAxis=+Y  TranslationCartesianOffset=[0 0 0]  TranslationROffset=0  TranslationROffsetUnits=m  TranslationZOffset=0  TranslationZOffsetUnits=m  TranslationThetaOffset=0  TranslationThetaOffsetUnits=deg  RotationMethod=StandardAxis  RotationAngleUnits=deg  RotationStandardAxis=-Y  RotationAngle=20  RotationArbitraryAxis=[0 0 1]  FollAlignAxisA=+X  BaseAlignAxisA=+Y  FollAlignAxisB=+Y  BaseAlignAxisB=+Z  RotationSequenceAxes=FollowerAxes  RotationSequence=XYX  RotationSequenceAngles=[0 0 0]  RotationSequenceAnglesUnits=deg  RotationMatrix=[1 0 0; 0 1 0; 0 0 1]
  Rigid Transform8 : sm_lib/Frames and Transforms/Rigid Transform  TranslationMethod=None  TranslationStandardOffset=-10  TranslationLengthUnit=m  TranslationStandardAxis=+Y  TranslationCartesianOffset=[0 0 0]  TranslationROffset=0  TranslationROffsetUnits=m  TranslationZOffset=0  TranslationZOffsetUnits=m  TranslationThetaOffset=0  TranslationThetaOffsetUnits=deg  RotationMethod=StandardAxis  RotationAngleUnits=deg  RotationStandardAxis=+Y  RotationAngle=20  RotationArbitraryAxis=[0 0 1]  FollAlignAxisA=+X  BaseAlignAxisA=+Y  FollAlignAxisB=+Y  BaseAlignAxisB=+Z  RotationSequenceAxes=FollowerAxes  RotationSequence=XYX  RotationSequenceAngles=[0 0 0]  RotationSequenceAnglesUnits=deg  RotationMatrix=[1 0 0; 0 1 0; 0 0 1]
  Rigid Transform9 : sm_lib/Frames and Transforms/Rigid Transform  TranslationMethod=Cartesian  TranslationStandardOffset=-10  TranslationLengthUnit=m  TranslationStandardAxis=+X  TranslationCartesianOffset=[-10 -10 10]  TranslationROffset=0  TranslationROffsetUnits=m  TranslationZOffset=0  TranslationZOffsetUnits=m  TranslationThetaOffset=0  TranslationThetaOffsetUnits=deg  RotationMethod=None  RotationAngleUnits=deg  RotationStandardAxis=+Z  RotationAngle=0.0  RotationArbitraryAxis=[0 0 1]  FollAlignAxisA=+X  BaseAlignAxisA=+Y  FollAlignAxisB=+Y  BaseAlignAxisB=+Z  RotationSequenceAxes=FollowerAxes  RotationSequence=XYX  RotationSequenceAngles=[0 0 0]  RotationSequenceAnglesUnits=deg  RotationMatrix=[1 0 0; 0 1 0; 0 0 1]
  Solver Configuration : nesl_utility/Solver Configuration  PhysicalDomain=network_engine_domain  SubClassName=solver  LeftPortType=input  RightPortType=generic  Tones=[]  Harmonics=[]  SimulateNoise=off  Profile=off  UseLocalSampling=off  EnableSwitchedLinearOptims=on  FrequencyDomain=off  UseCCode=off  RelTol=0.001  AbsTol=1e-06  MinStep=1e-09  ToWorkspace=off  RevertToSquareIcSolve=off  NumHomotopyIterations=100  PhasorMode=off  PhasorModeNumHarmonics=1  DoDC=off  ResidualTolerance=1e-9  UseLocalSolver=off  LocalSolverChoice=NE_BACKWARD_EULER_ADVANCER  LocalSolverSampleTime=.001  DoFixedCost=off  MaxNonlinIter=5  MaxModeIter=2  ComputeImpulses=off  ImpulseIterations=2  LinearAlgebra=Sparse  EquationFormulation=NE_TIME_EF  DelaysMemoryBudget=1024  AutomaticFiltering=on  FilteringTimeConstant=0.001  PartitionStorageMethod=AS_NEEDED  PartitionMemoryBudget=1024  PartitionMethod=FAST
      settings: SourceProductBaseCode=PW,SS
  SteeringFL : Subsystem
      settings: PortSchema="{\"entries\":[{\"content\":{\"sides\":[{\"content\":{\"connectorIds\":[\"LConn1\",\"Out1\"]},\"type\":\"ConnectorPlacement.EquallySpacedRectSide\",\"uuid\":\"aecb93a2-0be2-467a-815e-d47a1d9c337a\"},{\"content\":{\"connectorIds\":[\"In1\",\"RConn1\"],\"side\":\"RIGHT\"},\"type\":\"ConnectorPlacement.EquallySpacedRectSide\",\"uuid\":\"2e301024-cdba-4fce-ad7b-38681e5bd639\"},{\"content\":{\"connectorIds\":[],\"side\":\"TOP\"},\"type\":\"ConnectorPlacement.EquallySpacedRectSide\",\"uuid\":\"e5c8365e-8bdc-4a72-941e-2bfb1b04b607\"}]},\"type\":\"ConnectorPlacement.EquallySpacedConnector\",\"uuid\":\"9e86bc63-46c1-4c85-ad30-43b16503eba0\"}],\"packageUris\":[\"http://schema.mathworks.com/mf0/Connector/R2020b\"],\"version\":\"1.0\"}"
  SteeringFR : Subsystem
      settings: PortSchema="{\"entries\":[{\"content\":{\"sides\":[{\"content\":{\"connectorIds\":[\"LConn1\",\"Out1\"]},\"type\":\"ConnectorPlacement.EquallySpacedRectSide\",\"uuid\":\"aecb93a2-0be2-467a-815e-d47a1d9c337a\"},{\"content\":{\"connectorIds\":[\"In1\",\"RConn1\"],\"side\":\"RIGHT\"},\"type\":\"ConnectorPlacement.EquallySpacedRectSide\",\"uuid\":\"2e301024-cdba-4fce-ad7b-38681e5bd639\"},{\"content\":{\"connectorIds\":[],\"side\":\"TOP\"},\"type\":\"ConnectorPlacement.EquallySpacedRectSide\",\"uuid\":\"e5c8365e-8bdc-4a72-941e-2bfb1b04b607\"}]},\"type\":\"ConnectorPlacement.EquallySpacedConnector\",\"uuid\":\"9e86bc63-46c1-4c85-ad30-43b16503eba0\"}],\"packageUris\":[\"http://schema.mathworks.com/mf0/Connector/R2020b\"],\"version\":\"1.0\"}"
  SteeringRL : Subsystem
      settings: PortSchema="{\"entries\":[{\"content\":{\"sides\":[{\"content\":{\"connectorIds\":[\"LConn1\",\"Out1\"]},\"type\":\"ConnectorPlacement.EquallySpacedRectSide\",\"uuid\":\"aecb93a2-0be2-467a-815e-d47a1d9c337a\"},{\"content\":{\"connectorIds\":[\"In1\",\"RConn1\"],\"side\":\"RIGHT\"},\"type\":\"ConnectorPlacement.EquallySpacedRectSide\",\"uuid\":\"2e301024-cdba-4fce-ad7b-38681e5bd639\"},{\"content\":{\"connectorIds\":[],\"side\":\"TOP\"},\"type\":\"ConnectorPlacement.EquallySpacedRectSide\",\"uuid\":\"e5c8365e-8bdc-4a72-941e-2bfb1b04b607\"}]},\"type\":\"ConnectorPlacement.EquallySpacedConnector\",\"uuid\":\"9e86bc63-46c1-4c85-ad30-43b16503eba0\"}],\"packageUris\":[\"http://schema.mathworks.com/mf0/Connector/R2020b\"],\"version\":\"1.0\"}"
  SteeringRR : Subsystem
      settings: PortSchema="{\"entries\":[{\"content\":{\"sides\":[{\"content\":{\"connectorIds\":[\"LConn1\",\"Out1\"]},\"type\":\"ConnectorPlacement.EquallySpacedRectSide\",\"uuid\":\"aecb93a2-0be2-467a-815e-d47a1d9c337a\"},{\"content\":{\"connectorIds\":[\"In1\",\"RConn1\"],\"side\":\"RIGHT\"},\"type\":\"ConnectorPlacement.EquallySpacedRectSide\",\"uuid\":\"2e301024-cdba-4fce-ad7b-38681e5bd639\"},{\"content\":{\"connectorIds\":[],\"side\":\"TOP\"},\"type\":\"ConnectorPlacement.EquallySpacedRectSide\",\"uuid\":\"e5c8365e-8bdc-4a72-941e-2bfb1b04b607\"}]},\"type\":\"ConnectorPlacement.EquallySpacedConnector\",\"uuid\":\"9e86bc63-46c1-4c85-ad30-43b16503eba0\"}],\"packageUris\":[\"http://schema.mathworks.com/mf0/Connector/R2020b\"],\"version\":\"1.0\"}"
  Subsystem : Subsystem
  Subsystem6 : Subsystem
  Subsystem7 : Subsystem
  Subsystem8 : Subsystem
  "Transform XLines " : sm_lib/Frames and Transforms/Rigid Transform  TranslationMethod=Cartesian  TranslationStandardOffset=0  TranslationLengthUnit=m  TranslationStandardAxis=+Z  TranslationCartesianOffset=[0 0 0]  TranslationROffset=0  TranslationROffsetUnits=m  TranslationZOffset=0  TranslationZOffsetUnits=m  TranslationThetaOffset=0  TranslationThetaOffsetUnits=deg  RotationMethod=StandardAxis  RotationAngleUnits=deg  RotationStandardAxis=+Z  RotationAngle=90  RotationArbitraryAxis=[0 0 1]  FollAlignAxisA=+X  BaseAlignAxisA=+Y  FollAlignAxisB=+Y  BaseAlignAxisB=+Z  RotationSequenceAxes=FollowerAxes  RotationSequence=XYX  RotationSequenceAngles=[0 0 0]  RotationSequenceAnglesUnits=deg  RotationMatrix=[1 0 0; 0 1 0; 0 0 1]
  W->S : sm_lib/Frames and Transforms/Rigid Transform  TranslationMethod=Cartesian  TranslationStandardOffset=0  TranslationLengthUnit=m  TranslationStandardAxis=+Z  TranslationCartesianOffset=[500.0 0 0.350+0.100]  TranslationROffset=0  TranslationROffsetUnits=m  TranslationZOffset=0  TranslationZOffsetUnits=m  TranslationThetaOffset=0  TranslationThetaOffsetUnits=deg  RotationMethod=None  RotationAngleUnits=deg  RotationStandardAxis=+Z  RotationAngle=0.0  RotationArbitraryAxis=[0 0 1]  FollAlignAxisA=+X  BaseAlignAxisA=+Y  FollAlignAxisB=+Y  BaseAlignAxisB=+Z  RotationSequenceAxes=FollowerAxes  RotationSequence=XYX  RotationSequenceAngles=[0 0 0]  RotationSequenceAnglesUnits=deg  RotationMatrix=[1 0 0; 0 1 0; 0 0 1]
  W->S1 : sm_lib/Frames and Transforms/Rigid Transform  TranslationMethod=Cartesian  TranslationStandardOffset=0  TranslationLengthUnit=m  TranslationStandardAxis=+Z  TranslationCartesianOffset=[500.0 0 0.]  TranslationROffset=0  TranslationROffsetUnits=m  TranslationZOffset=0  TranslationZOffsetUnits=m  TranslationThetaOffset=0  TranslationThetaOffsetUnits=deg  RotationMethod=None  RotationAngleUnits=deg  RotationStandardAxis=+Z  RotationAngle=0.0  RotationArbitraryAxis=[0 0 1]  FollAlignAxisA=+X  BaseAlignAxisA=+Y  FollAlignAxisB=+Y  BaseAlignAxisB=+Z  RotationSequenceAxes=FollowerAxes  RotationSequence=XYX  RotationSequenceAngles=[0 0 0]  RotationSequenceAnglesUnits=deg  RotationMatrix=[1 0 0; 0 1 0; 0 0 1]
  WFL_kinematic_quantities : Subsystem
      settings: PortSchema="{\"entries\":[{\"content\":{\"sides\":[{\"content\":{\"connectorIds\":[\"In1\",\"In2\",\"In3\"]},\"type\":\"ConnectorPlacement.EquallySpacedRectSide\",\"uuid\":\"ec47a64e-a5fd-4633-80db-b84bba5d7902\"},{\"content\":{\"connectorIds\":[],\"side\":\"RIGHT\"},\"type\":\"ConnectorPlacement.EquallySpacedRectSide\",\"uuid\":\"3d46d3c3-244c-4d8e-b3dc-417a724bf33d\"},{\"content\":{\"connectorIds\":[\"LConn1\",\"LConn2\"],\"side\":\"TOP\"},\"type\":\"ConnectorPlacement.EquallySpacedRectSide\",\"uuid\":\"f20a4a76-81c8-4cc3-9c31-331f4e6b9dce\"}]},\"type\":\"ConnectorPlacement.EquallySpacedConnector\",\"uuid\":\"9b7cd881-f254-4da0-bdfb-8b1718d855b4\"}],\"packageUris\":[\"http://schema.mathworks.com/mf0/Connector/R2020b\"],\"version\":\"1.0\"}"
  WFR_kinematic_quantities : Subsystem
      settings: PortSchema="{\"entries\":[{\"content\":{\"sides\":[{\"content\":{\"connectorIds\":[\"In1\",\"In2\",\"In3\"]},\"type\":\"ConnectorPlacement.EquallySpacedRectSide\",\"uuid\":\"ec47a64e-a5fd-4633-80db-b84bba5d7902\"},{\"content\":{\"connectorIds\":[],\"side\":\"RIGHT\"},\"type\":\"ConnectorPlacement.EquallySpacedRectSide\",\"uuid\":\"3d46d3c3-244c-4d8e-b3dc-417a724bf33d\"},{\"content\":{\"connectorIds\":[\"LConn1\",\"LConn2\"],\"side\":\"TOP\"},\"type\":\"ConnectorPlacement.EquallySpacedRectSide\",\"uuid\":\"f20a4a76-81c8-4cc3-9c31-331f4e6b9dce\"}]},\"type\":\"ConnectorPlacement.EquallySpacedConnector\",\"uuid\":\"9b7cd881-f254-4da0-bdfb-8b1718d855b4\"}],\"packageUris\":[\"http://schema.mathworks.com/mf0/Connector/R2020b\"],\"version\":\"1.0\"}"
  WRL_kinematic_quantities : Subsystem
      settings: PortSchema="{\"entries\":[{\"content\":{\"sides\":[{\"content\":{\"connectorIds\":[\"In1\",\"In2\",\"In3\"]},\"type\":\"ConnectorPlacement.EquallySpacedRectSide\",\"uuid\":\"ec47a64e-a5fd-4633-80db-b84bba5d7902\"},{\"content\":{\"connectorIds\":[],\"side\":\"RIGHT\"},\"type\":\"ConnectorPlacement.EquallySpacedRectSide\",\"uuid\":\"3d46d3c3-244c-4d8e-b3dc-417a724bf33d\"},{\"content\":{\"connectorIds\":[\"LConn1\",\"LConn2\"],\"side\":\"TOP\"},\"type\":\"ConnectorPlacement.EquallySpacedRectSide\",\"uuid\":\"f20a4a76-81c8-4cc3-9c31-331f4e6b9dce\"}]},\"type\":\"ConnectorPlacement.EquallySpacedConnector\",\"uuid\":\"9b7cd881-f254-4da0-bdfb-8b1718d855b4\"}],\"packageUris\":[\"http://schema.mathworks.com/mf0/Connector/R2020b\"],\"version\":\"1.0\"}"
  WRR_kinematic_quantities : Subsystem
      settings: PortSchema="{\"entries\":[{\"content\":{\"sides\":[{\"content\":{\"connectorIds\":[\"In1\",\"In2\",\"In3\"]},\"type\":\"ConnectorPlacement.EquallySpacedRectSide\",\"uuid\":\"ec47a64e-a5fd-4633-80db-b84bba5d7902\"},{\"content\":{\"connectorIds\":[],\"side\":\"RIGHT\"},\"type\":\"ConnectorPlacement.EquallySpacedRectSide\",\"uuid\":\"3d46d3c3-244c-4d8e-b3dc-417a724bf33d\"},{\"content\":{\"connectorIds\":[\"LConn1\",\"LConn2\"],\"side\":\"TOP\"},\"type\":\"ConnectorPlacement.EquallySpacedRectSide\",\"uuid\":\"f20a4a76-81c8-4cc3-9c31-331f4e6b9dce\"}]},\"type\":\"ConnectorPlacement.EquallySpacedConnector\",\"uuid\":\"9b7cd881-f254-4da0-bdfb-8b1718d855b4\"}],\"packageUris\":[\"http://schema.mathworks.com/mf0/Connector/R2020b\"],\"version\":\"1.0\"}"
  World Frame : sm_lib/Frames and Transforms/World Frame
  calc_VC_from_meas : Subsystem
  calc_betaC_from_meas : Subsystem
  get_measurements : Subsystem
      settings: PortSchema="{\"entries\":[{\"content\":{\"sides\":[{\"content\":{\"connectorIds\":[\"LConn1\"]},\"type\":\"ConnectorPlacement.EquallySpacedRectSide\",\"uuid\":\"391bc4a3-95a3-452b-a808-542cf1893521\"},{\"content\":{\"connectorIds\":[\"Out1\",\"Out2\",\"Out3\",\"Out4\",\"Out5\",\"Out6\"],\"side\":\"RIGHT\"},\"type\":\"ConnectorPlacement.EquallySpacedRectSide\",\"uuid\":\"9b13380a-f379-4ce9-a7fd-32629b87c6ba\"},{\"content\":{\"connectorIds\":[\"LConn2\"],\"side\":\"TOP\"},\"type\":\"ConnectorPlacement.EquallySpacedRectSide\",\"uuid\":\"05d317f5-3845-49c9-be0f-44f8dd6fefcb\"}]},\"type\":\"ConnectorPlacement.EquallySpacedConnector\",\"uuid\":\"1e13e943-51f4-4bc8-a8df-e45759fa434f\"}],\"packageUris\":[\"http://schema.mathworks.com/mf0/Connector/R2020b\"],\"version\":\"1.0\"}"
  meas_FLwheel_kinematic_quantities_in_Simscape : Subsystem
      settings: PortSchema="{\"entries\":[{\"content\":{\"sides\":[{\"content\":{\"connectorIds\":[\"LConn1\"]},\"type\":\"ConnectorPlacement.EquallySpacedRectSide\",\"uuid\":\"e03321fd-25bb-4819-9f1e-db734f4e967c\"},{\"content\":{\"connectorIds\":[\"Out1\"],\"side\":\"RIGHT\"},\"type\":\"ConnectorPlacement.EquallySpacedRectSide\",\"uuid\":\"050ab202-eafa-442c-9986-79063696eccf\"},{\"content\":{\"connectorIds\":[\"LConn2\",\"LConn3\"],\"side\":\"TOP\"},\"type\":\"ConnectorPlacement.EquallySpacedRectSide\",\"uuid\":\"8dcced68-89d3-4768-b866-17e377279429\"}]},\"type\":\"ConnectorPlacement.EquallySpacedConnector\",\"uuid\":\"0bf22017-ba9a-4fa7-bda6-31ede33e3ebb\"}],\"packageUris\":[\"http://schema.mathworks.com/mf0/Connector/R2020b\"],\"version\":\"1.0\"}"
  meas_FRwheel_kinematic_quantities_in_Simscape : Subsystem
      settings: PortSchema="{\"entries\":[{\"content\":{\"sides\":[{\"content\":{\"connectorIds\":[\"LConn1\"]},\"type\":\"ConnectorPlacement.EquallySpacedRectSide\",\"uuid\":\"e03321fd-25bb-4819-9f1e-db734f4e967c\"},{\"content\":{\"connectorIds\":[\"Out1\"],\"side\":\"RIGHT\"},\"type\":\"ConnectorPlacement.EquallySpacedRectSide\",\"uuid\":\"050ab202-eafa-442c-9986-79063696eccf\"},{\"content\":{\"connectorIds\":[\"LConn2\",\"LConn3\"],\"side\":\"TOP\"},\"type\":\"ConnectorPlacement.EquallySpacedRectSide\",\"uuid\":\"8dcced68-89d3-4768-b866-17e377279429\"}]},\"type\":\"ConnectorPlacement.EquallySpacedConnector\",\"uuid\":\"0bf22017-ba9a-4fa7-bda6-31ede33e3ebb\"}],\"packageUris\":[\"http://schema.mathworks.com/mf0/Connector/R2020b\"],\"version\":\"1.0\"}"
  meas_RLwheel_kinematic_quantities_in_Simscape : Subsystem
      settings: PortSchema="{\"entries\":[{\"content\":{\"sides\":[{\"content\":{\"connectorIds\":[\"LConn1\"]},\"type\":\"ConnectorPlacement.EquallySpacedRectSide\",\"uuid\":\"e03321fd-25bb-4819-9f1e-db734f4e967c\"},{\"content\":{\"connectorIds\":[\"Out1\"],\"side\":\"RIGHT\"},\"type\":\"ConnectorPlacement.EquallySpacedRectSide\",\"uuid\":\"050ab202-eafa-442c-9986-79063696eccf\"},{\"content\":{\"connectorIds\":[\"LConn2\",\"LConn3\"],\"side\":\"TOP\"},\"type\":\"ConnectorPlacement.EquallySpacedRectSide\",\"uuid\":\"8dcced68-89d3-4768-b866-17e377279429\"}]},\"type\":\"ConnectorPlacement.EquallySpacedConnector\",\"uuid\":\"0bf22017-ba9a-4fa7-bda6-31ede33e3ebb\"}],\"packageUris\":[\"http://schema.mathworks.com/mf0/Connector/R2020b\"],\"version\":\"1.0\"}"
  meas_RRwheel_kinematic_quantities_in_Simscape : Subsystem
      settings: PortSchema="{\"entries\":[{\"content\":{\"sides\":[{\"content\":{\"connectorIds\":[\"LConn1\"]},\"type\":\"ConnectorPlacement.EquallySpacedRectSide\",\"uuid\":\"e03321fd-25bb-4819-9f1e-db734f4e967c\"},{\"content\":{\"connectorIds\":[\"Out1\"],\"side\":\"RIGHT\"},\"type\":\"ConnectorPlacement.EquallySpacedRectSide\",\"uuid\":\"050ab202-eafa-442c-9986-79063696eccf\"},{\"content\":{\"connectorIds\":[\"LConn2\",\"LConn3\"],\"side\":\"TOP\"},\"type\":\"ConnectorPlacement.EquallySpacedRectSide\",\"uuid\":\"8dcced68-89d3-4768-b866-17e377279429\"}]},\"type\":\"ConnectorPlacement.EquallySpacedConnector\",\"uuid\":\"0bf22017-ba9a-4fa7-bda6-31ede33e3ebb\"}],\"packageUris\":[\"http://schema.mathworks.com/mf0/Connector/R2020b\"],\"version\":\"1.0\"}"
  Meas : Outport
  Fz : Outport  Port=2
  fcx_SS : Outport  Port=3
  wires:
  [VCy_meas] -> calc_VC_from_meas/2(VCy_meas)
  [RL_kin] -> WRL_kinematic_quantities/2(RL_kin)
  [VCx_meas] -> calc_VC_from_meas/1(VCx_meas)
  meas_FRwheel_kinematic_quantities_in_Simscape/1(FR_kin) -> [FR_kin]
  [deltaRR_meas] -> Bus Creator1/15  "deltaRR_meas"
  [RR_kin] -> WRR_kinematic_quantities/2(RR_kin)
  [MayRL_cmd] -> WRL_kinematic_quantities/3(MyaRL)
  [FzRR] -> WRR_kinematic_quantities/1(FzRR_meas)
  GroundReactionRL/1(fzRL) -> [FzRL]
  get_measurements/4(dPsi_meas) -> [dPsi_meas]
  [VCy_meas] -> calc_betaC_from_meas/1(VCy_meas)
  [deltaFR_meas] -> Bus Creator1/14  "deltaFR_meas"
  get_measurements/6(VCy_meas) -> [VCy_meas]
  [FzFL] -> WFL_kinematic_quantities/1(FzFL_meas)
  calc_betaC_from_meas/1(betaC_meas) -> [betaC_meas]
  [FL_kin] -> WFL_kinematic_quantities/2(FL_kin)
  get_measurements/5(VCx_meas) -> [VCx_meas]
  [VCx_meas] -> calc_betaC_from_meas/2(VCx_meas)
  calc_VC_from_meas/1(VC_meas) -> [VC_meas]
  [deltaRL_meas] -> Bus Creator1/16  "deltaRL_meas"
  [FR_kin] -> WFR_kinematic_quantities/2(FR_kin)
  [MayRR_cmd] -> WRR_kinematic_quantities/3(MyaRR)
  [deltaFL_meas] -> Bus Creator1/13  "deltaFL_meas"
  meas_FLwheel_kinematic_quantities_in_Simscape/1(FL_kin) -> [FL_kin]
  [FzRL] -> WRL_kinematic_quantities/1(FzRL_meas)
  [FzFR] -> WFR_kinematic_quantities/1(FzFR_meas)
  [MayFR_cmd] -> WFR_kinematic_quantities/3(MyaFR)
  meas_RLwheel_kinematic_quantities_in_Simscape/1(RL_kin) -> [RL_kin]
  meas_RRwheel_kinematic_quantities_in_Simscape/1(RR_kin) -> [RR_kin]
  delta_cmd/1 -> Bus Selector/1
  Bus Selector/1 -> [deltaFL_cmd]  "<deltaFL_cmd>"
  [betaC_meas] -> Bus Creator1/4  "betaC_meas"
  Bus Selector/2 -> [deltaFR_cmd]  "<deltaFR_cmd>"
  Bus Selector/3 -> [deltaRR_cmd]  "<deltaRR_cmd>"
  Bus Selector/4 -> [deltaRL_cmd]  "<deltaRL_cmd>"
  May_cmd/1 -> Bus Selector1/1
  [dPsi_meas] -> Bus Creator1/8  "dPsi_meas"
  get_measurements/1(Theta_meas) -> [Theta_meas]
  [Psi_meas] -> Bus Creator1/7  "Psi_meas"
  [VC_meas] -> Bus Creator1/1  "VC_meas"
  Bus Creator1/1 -> [measurements]
  [FR_kin] -> Bus Selector3/1
  Bus Selector3/1 -> [dOmegaFR_meas]  "<dOmegaFR_meas>"
  Bus Selector4/1 -> [dOmegaFL_meas]  "<dOmegaFL_meas>"
  [FL_kin] -> Bus Selector4/1
  Bus Selector5/1 -> [dOmegaRR_meas]  "<dOmegaRR_meas>"
  [RR_kin] -> Bus Selector5/1
  [RL_kin] -> Bus Selector6/1
  Bus Selector6/1 -> [dOmegaRL_meas]  "<dOmegaRL_meas>"
  [dOmegaFR_meas] -> Bus Creator1/10  "dOmegaFR_meas"
  [dOmegaFL_meas] -> Bus Creator1/9  "dOmegaFL_meas"
  [dOmegaRR_meas] -> Bus Creator1/11  "dOmegaRR_meas"
  [dOmegaRL_meas] -> Bus Creator1/12  "dOmegaRL_meas"
  [measurements] -> Meas/1
  SteeringRL/1(deltaRL_meas) -> [deltaRL_meas]
  [deltaFL_cmd] -> SteeringFL/1(deltaFL_cmd)
  SteeringFL/1(deltaFL_meas) -> [deltaFL_meas]
  GroundReactionFL/1(FzFL) -> [FzFL]
  GroundReactionRR/1(fzRR) -> [FzRR]
  [deltaRR_cmd] -> SteeringRR/1(deltaRR_cmd)
  SteeringRR/1(deltaRR_meas) -> [deltaRR_meas]
  GroundReactionFR/1(fzFR) -> [FzFR]
  SteeringFR/1(deltaFR_meas) -> [deltaFR_meas]
  [deltaFR_cmd] -> SteeringFR/1(deltaFR_cmd)
  [deltaRL_cmd] -> SteeringRL/1(deltaRL_cmd)
  [FzFL] -> Bus Creator/1  "FzFL"
  [FzFR] -> Bus Creator/2  "FzFR"
  [FzRR] -> Bus Creator/3  "FzRR"
  [FzRL] -> Bus Creator/4  "FzRL"
  Bus Creator/1 -> [Fz]
  [Fz] -> Fz/1
  get_measurements/2(Phi_meas) -> [Phi_meas]
  get_measurements/3(Psi_meas) -> [Psi_meas]
  [Phi_meas] -> Bus Creator1/6  "Phi_meas"
  [Theta_meas] -> Bus Creator1/5  "Theta_meas"
  [MayFL_cmd] -> WFL_kinematic_quantities/3(MyaFL)
  Bus Selector1/1 -> [MayFL_cmd]  "<MayFL_cmd>"
  Bus Selector1/2 -> [MayFR_cmd]  "<MayFR_cmd>"
  Bus Selector1/3 -> [MayRR_cmd]  "<MayRR_cmd>"
  Bus Selector1/4 -> [MayRL_cmd]  "<MayRL_cmd>"
  [VCx_meas] -> Bus Creator1/2  "VCx_meas"
  [VCy_meas] -> Bus Creator1/3  "VCy_meas"
  xi_cmd/1 -> Bus Selector2/1
  Bus Selector2/1 -> [Theta1_cmd]  "<Theta1_cmd>"
  Bus Selector2/2 -> [Theta2_cmd]  "<Theta2_cmd>"
  Bus Selector2/3 -> [x3_cmd]  "<x3_cmd>"
  [Theta1_cmd] -> "Hydraulic manipulator, Simscape"/1(Theta1 [rad])
  [Theta2_cmd] -> "Hydraulic manipulator, Simscape"/2(Theta2 [rad])
  [x3_cmd] -> "Hydraulic manipulator, Simscape"/3(x3[m])
  "Hydraulic manipulator, Simscape"/1(fcx_SS) -> [fcx_SS]
  [fcx_SS] -> fcx_SS/1
  connections:
  Connection Label/LConn1 -- Chassis frames/LConn1
  Connection Label11/LConn1 -- Subsystem/LConn1
  Chassis frames/RConn2 -- Connection Label18/LConn1
  Connection Label28/LConn1 -- W->S/RConn1
  Bushing Joint/RConn1 -- Connection Label21/LConn1
  GroundReactionRL/RConn1 -- Connection Label40/LConn1
  Connection Label75/LConn1 -- Chassis frames/RConn4
  Connection Label52/LConn1 -- WRR_kinematic_quantities/LConn1
  Connection Label63/LConn1 -- get_measurements/LConn1
  Connection Label10/LConn1 -- ActuationRL/LConn1
  World Frame/RConn1 -- MechanismConfiguration/RConn1 -- Solver Configuration/RConn1 -- W->S1/LConn1 -- Connection Label23/LConn1 -- Floor/LConn1 -- W->S/LConn1
  Connection Label30/LConn1 -- meas_RLwheel_kinematic_quantities_in_Simscape/LConn2
  SteeringRL/LConn1 -- Connection Label6/LConn1
  Connection Label24/LConn1 -- Subsystem8/LConn1
  GroundReactionRL/RConn2 -- Connection Label39/LConn1
  Subsystem6/LConn1 -- Connection Label12/LConn1
  Connection Label27/LConn1 -- Subsystem7/LConn1
  Bushing Joint/LConn1 -- Connection Label22/LConn1
  Connection Label17/LConn1 -- Chassis frames/RConn1
  Connection Label29/LConn1 -- meas_RLwheel_kinematic_quantities_in_Simscape/LConn1
  Connection Label4/LConn1 -- Chassis frames/LConn2
  ActuationRL/RConn1 -- Connection Label9/LConn1
  Chassis frames/RConn3 -- Connection Label2/LConn1
  Connection Label49/LConn1 -- WFL_kinematic_quantities/LConn2
  Connection Label48/LConn1 -- WFL_kinematic_quantities/LConn1
  Connection Label57/LConn1 -- meas_FRwheel_kinematic_quantities_in_Simscape/LConn2
  Connection Label65/LConn1 -- meas_FRwheel_kinematic_quantities_in_Simscape/LConn3
  Connection Label53/LConn1 -- WRR_kinematic_quantities/LConn2
  Connection Label36/LConn1 -- WFR_kinematic_quantities/LConn2
  Connection Label59/LConn1 -- get_measurements/LConn2
  Connection Label51/LConn1 -- WRL_kinematic_quantities/LConn2
  Connection Label50/LConn1 -- WRL_kinematic_quantities/LConn1
  Connection Label46/LConn1 -- meas_FLwheel_kinematic_quantities_in_Simscape/LConn2
  Connection Label47/LConn1 -- meas_FLwheel_kinematic_quantities_in_Simscape/LConn3
  Connection Label45/LConn1 -- meas_FLwheel_kinematic_quantities_in_Simscape/LConn1
  Connection Label31/LConn1 -- meas_RLwheel_kinematic_quantities_in_Simscape/LConn3
  Connection Label56/LConn1 -- meas_FRwheel_kinematic_quantities_in_Simscape/LConn1
  Connection Label35/LConn1 -- WFR_kinematic_quantities/LConn1
  Connection Label32/LConn1 -- meas_RRwheel_kinematic_quantities_in_Simscape/LConn1
  Connection Label33/LConn1 -- meas_RRwheel_kinematic_quantities_in_Simscape/LConn2
  Connection Label34/LConn1 -- meas_RRwheel_kinematic_quantities_in_Simscape/LConn3
  SteeringFL/LConn1 -- Connection Label5/LConn1
  Connection Label1/LConn1 -- SteeringFL/RConn1
  Connection Label7/LConn1 -- ActuationFL/LConn1
  ActuationFL/RConn1 -- Connection Label8/LConn1
  GroundReactionFL/RConn1 -- Connection Label55/LConn1
  GroundReactionFL/RConn2 -- Connection Label54/LConn1
  Connection Label43/LConn1 -- ActuationRR/LConn1
  ActuationRR/RConn1 -- Connection Label44/LConn1
  SteeringRR/LConn1 -- Connection Label26/LConn1
  Connection Label25/LConn1 -- SteeringRR/RConn1
  GroundReactionFR/RConn2 -- Connection Label13/LConn1
  GroundReactionFR/RConn1 -- Connection Label14/LConn1
  SteeringFR/LConn1 -- Connection Label16/LConn1
  Connection Label15/LConn1 -- SteeringFR/RConn1
  ActuationFR/RConn1 -- Connection Label42/LConn1
  Connection Label41/LConn1 -- ActuationFR/LConn1
  Connection Label38/LConn1 -- GroundReactionRR/RConn1
  Connection Label37/LConn1 -- GroundReactionRR/RConn2
  Connection Label3/LConn1 -- SteeringRL/RConn1
  Connection Label19/LConn1 -- Chassis frames/RConn5
  Rigid Transform/LConn1 -- Connection Label20/LConn1
  Rigid Transform/RConn1 -- Connection Label58/LConn1
  Rigid Transform1/LConn1 -- Connection Label60/LConn1
  Connection Label62/LConn1 -- Rigid Transform1/RConn1
  Connection Label67/LConn1 -- "Hydraulic manipulator, Simscape"/LConn1
  Connection Label64/LConn1 -- Rigid Transform2/LConn1 -- Rigid Transform9/LConn1 -- Rigid Transform4/LConn1 -- Rigid Transform3/LConn1
  Floor Grid 2/RConn1 -- "Transform XLines "/RConn1
  "Transform XLines "/LConn1 -- W->S1/RConn1 -- Floor Grid 1/RConn1
  Rigid Transform5/LConn1 -- Rigid Transform4/RConn1
  Rigid Transform6/LConn1 -- Rigid Transform5/RConn1
  Rigid Transform6/RConn1 -- Camera2/RConn1
  Rigid Transform7/LConn1 -- Rigid Transform2/RConn1
  Rigid Transform7/RConn1 -- Camera0/RConn1
  Rigid Transform8/LConn1 -- Rigid Transform3/RConn1
  Rigid Transform8/RConn1 -- Camera1/RConn1
  Rigid Transform11/RConn1 -- Camera3/RConn1
  Rigid Transform10/LConn1 -- Rigid Transform9/RConn1
  Rigid Transform11/LConn1 -- Rigid Transform10/RConn1
